simulink model "mmcontrollerVerification_th"  (R2018b)
settings: Solver=ode15s  StartTime=0.0  StopTime=duration_s  MaxStep=5  RelTol=1e-3  AbsTol=1e-3
values from neighbouring files (symbols this model uses):
  ini_euler_ang = [0;ini_pitch;0]    [mmcontrollerVerification_ts.m]
  ini_O_Vcm_o = [0;0;0.0]    [mmcontrollerVerification_ts.m]
  ini_Rcm_o = ini_Rcm_o    [mmcontrollerVerification_ts.m]
undefined symbols (not defined in the file or in its folder): gnd_station, ini_OwB, ini_platform_ang, ini_platform_vel, maxWinchAccel, maxWinchSpeed, R11_g, R1n_cm, R21_g, R2n_cm, R31_g, R3n_cm, rotation_sequence, sim_param, unstretched_l
libraries: thrAttachPtKinematics_ul x6, singleTetherNGreater2_cl x3, winch_ul x3, vrlib x3, eulAng2RotMat_ul x2, combinedController_cl x1, simulink x1, massSpringDamper_ul x1
settings Model: Creator=mcobb  LastModifiedBy=asiddiq2

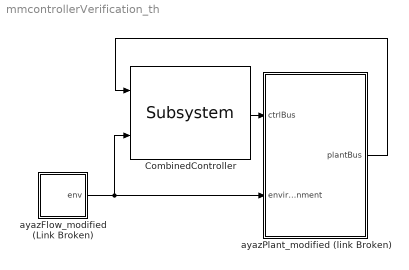
== system mmcontrollerVerification_th ==
  CombinedController : combinedController_cl/Subsystem  a_user=0  b_user=0  phiG_user=0  path_user=0  S_user=0
  ayazFlow_modified (Link Broken) : Subsystem
  ayazPlant_modified (link Broken) : Subsystem
  wires:
  CombinedController/1 -> ayazPlant_modified (link Broken)/1(ctrlBus)
  ayazPlant_modified (link Broken)/1(plantBus) -> CombinedController/1
  ayazFlow_modified (Link Broken)/1(env) -> CombinedController/2, ayazPlant_modified (link Broken)/2(environment)

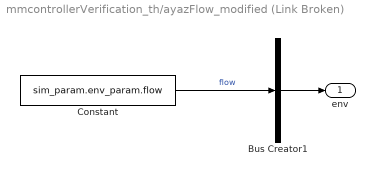
== system mmcontrollerVerification_th/ayazFlow_modified (Link Broken) ==
  Bus Creator1 : BusCreator  Inputs=1  OutDataTypeStr=Bus: envBus
  Constant : Constant  Value=sim_param.env_param.flow
  env : Outport  OutDataTypeStr=Bus: envBus
  wires:
  Constant/1 -> Bus Creator1/1  "flow"
  Bus Creator1/1 -> env/1

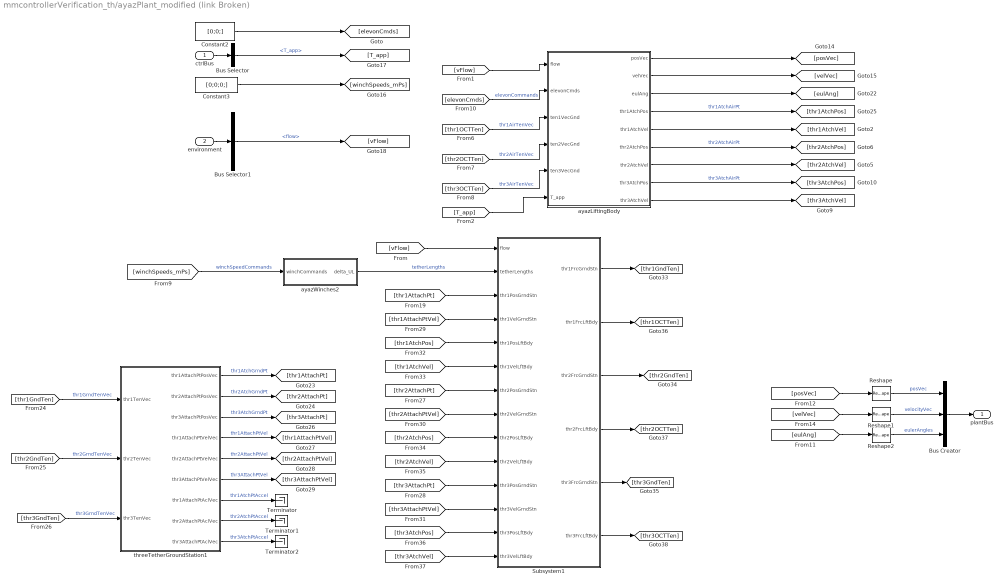
== system mmcontrollerVerification_th/ayazPlant_modified (link Broken) ==
  ctrlBus : Inport  OutDataTypeStr=Bus: ctrlBus
  environment : Inport  Port=2  OutDataTypeStr=Bus: envBus
  Bus Creator : BusCreator  Inputs=3  OutDataTypeStr=Bus: plantBus
  Bus Selector : BusSelector  OutputSignals=T_app
  Bus Selector1 : BusSelector  OutputSignals=flow
  Constant2 : Constant  Value=[0;0;]
  Constant3 : Constant  Value=[0;0;0;]
  Reshape : Reshape  OutputDimensionality=Column vector (2-D)
  Reshape1 : Reshape  OutputDimensionality=Column vector (2-D)
  Reshape2 : Reshape  OutputDimensionality=Column vector (2-D)
  Subsystem1 : Subsystem
  Terminator : Terminator
  Terminator1 : Terminator
  Terminator2 : Terminator
  ayazLiftingBody : Subsystem
  ayazWinches2 : Subsystem  mask{maxSpeed=maxWinchSpeed, maxAccel=maxWinchAccel, timeConst=1, tetherLengths=unstretched_l}
      mask prompts: maxSpeed "Winch Max Speed"; maxAccel "Winch Max Acceleration"; timeConst "Winch Time Constant"; tetherLengths "Initial tether lengths"
  threeTetherGroundStation1 : Subsystem  mask{fixed=1, J=sim_param.platform_param.platform_Izz, b=sim_param.platform_param.platform_damping, posVec=[0 0 0], thr1AttachPt=sim_param.tether_imp_nodes.R11_g, thr2AttachPt=sim_param.tether_imp_nodes.R21_g, thr3AttachPt=sim_param.tether_imp_nodes.R31_g, initAngPos=ini_platform_ang, initAngVel=ini_platform_vel}
      mask prompts: fixed "Free Spin Enable (==0 -> No Rotation, ~=0 -> Free Spinning)"; J "Rotational Inertia"; b "Damping coefficient"; posVec "Position Vector"; thr1AttachPt "Tether 1"; thr2AttachPt "Tether 2"; thr3AttachPt "Tether 3"; initAngPos "Initial angle"; initAngVel "Inital angular velocity"
      mask DialogControl Container5 Prompt: Physical Parameters
      mask DialogControl Container3 Prompt: Tether attachment position vectors: platform frame
      mask DialogControl Container4 Prompt: Initial conditions
  plantBus : Outport  OutDataTypeStr=Bus: plantBus
  wires:
  [eulAng] -> Reshape2/1
  [velVec] -> Reshape1/1
  [posVec] -> Reshape/1
  Subsystem1/5(thr3FrcGrndStn) -> [thr3GndTen]
  Subsystem1/6(thr3FrcLftBdy) -> [thr3OCTTen]
  Subsystem1/4(thr2FrcLftBdy) -> [thr2OCTTen]
  Subsystem1/3(thr2FrcGrndStn) -> [thr2GndTen]
  Subsystem1/2(thr1FrcLftBdy) -> [thr1OCTTen]
  Subsystem1/1(thr1FrcGrndStn) -> [thr1GndTen]
  [thr1AtchVel] -> Subsystem1/6(thr1VelLftBdy)
  [thr2AtchPos] -> Subsystem1/9(thr2PosLftBdy)
  [thr2AtchVel] -> Subsystem1/10(thr2VelLftBdy)
  [thr3AtchPos] -> Subsystem1/13(thr3PosLftBdy)
  [thr3AtchVel] -> Subsystem1/14(thr3VelLftBdy)
  [thr1AtchPos] -> Subsystem1/5(thr1PosLftBdy)
  [thr1AttachPtVel] -> Subsystem1/4(thr1VelGrndStn)
  [thr2AttachPtVel] -> Subsystem1/8(thr2VelGrndStn)
  [thr3AttachPtVel] -> Subsystem1/12(thr3VelGrndStn)
  [thr3AttachPt] -> Subsystem1/11(thr3PosGrndStn)
  [thr2AttachPt] -> Subsystem1/7(thr2PosGrndStn)
  [thr1AttachPt] -> Subsystem1/3(thr1PosGrndStn)
  [vFlow] -> Subsystem1/1(flow)
  threeTetherGroundStation1/7(thr1AttachPtAclVec) -> Terminator/1  "thr1AtchPtAccel"
  [thr1GndTen] -> threeTetherGroundStation1/1(thr1TenVec)  "thr1GrndTenVec"
  [thr3GndTen] -> threeTetherGroundStation1/3(thr3TenVec)  "thr3GrndTenVec"
  [winchSpeeds_mPs] -> ayazWinches2/1(winchCommands)  "winchSpeedCommands"
  [thr2GndTen] -> threeTetherGroundStation1/2(thr2TenVec)  "thr2GrndTenVec"
  ayazWinches2/1(delta_UL) -> Subsystem1/2(tetherLengths)  "tetherLengths"
  threeTetherGroundStation1/1(thr1AttachPtPosVec) -> [thr1AttachPt]  "thr1AtchGrndPt"
  threeTetherGroundStation1/3(thr3AttachPtPosVec) -> [thr3AttachPt]  "thr3AtchGrndPt"
  threeTetherGroundStation1/2(thr2AttachPtPosVec) -> [thr2AttachPt]  "thr2AtchGrndPt"
  threeTetherGroundStation1/4(thr1AttachPtVelVec) -> [thr1AttachPtVel]  "thr1AttachPtVel"
  threeTetherGroundStation1/8(thr2AttachPtAclVec) -> Terminator1/1  "thr2AtchPtAccel"
  threeTetherGroundStation1/5(thr2AttachPtVelVec) -> [thr2AttachPtVel]  "thr2AttachPtVel"
  threeTetherGroundStation1/6(thr3AttachPtVelVec) -> [thr3AttachPtVel]  "thr3AttachPtVel"
  threeTetherGroundStation1/9(thr3AttachPtAclVec) -> Terminator2/1  "thr3AtchPtAccel"
  ayazLiftingBody/9(thr3AtchVel) -> [thr3AtchVel]
  ayazLiftingBody/8(thr3AtchPos) -> [thr3AtchPos]  "thr3AtchAirPt"
  ayazLiftingBody/7(thr2AtchVel) -> [thr2AtchVel]
  ayazLiftingBody/6(thr2AtchPos) -> [thr2AtchPos]  "thr2AtchAirPt"
  ayazLiftingBody/5(thr1AtchVel) -> [thr1AtchVel]
  ayazLiftingBody/4(thr1AtchPos) -> [thr1AtchPos]  "thr1AtchAirPt"
  ayazLiftingBody/3(eulAng) -> [eulAng]
  Reshape1/1 -> Bus Creator/2  "velocityVec"
  Reshape2/1 -> Bus Creator/3  "eulerAngles"
  Reshape/1 -> Bus Creator/1  "posVec"
  Bus Creator/1 -> plantBus/1
  Bus Selector/1 -> [T_app]  "<T_app>"
  ctrlBus/1 -> Bus Selector/1
  environment/1 -> Bus Selector1/1
  [elevonCmds] -> ayazLiftingBody/2(elevonCmds)  "elevonCommands"
  [thr3OCTTen] -> ayazLiftingBody/5(ten3VecGnd)  "thr3AirTenVec"
  [thr2OCTTen] -> ayazLiftingBody/4(ten2VecGnd)  "thr2AirTenVec"
  [thr1OCTTen] -> ayazLiftingBody/3(ten1VecGnd)  "thr1AirTenVec"
  [vFlow] -> ayazLiftingBody/1(flow)
  ayazLiftingBody/2(velVec) -> [velVec]
  ayazLiftingBody/1("posVec ") -> [posVec]
  [T_app] -> ayazLiftingBody/6(T_app)
  Constant2/1 -> [elevonCmds]
  Constant3/1 -> [winchSpeeds_mPs]
  Bus Selector1/1 -> [vFlow]  "<flow>"

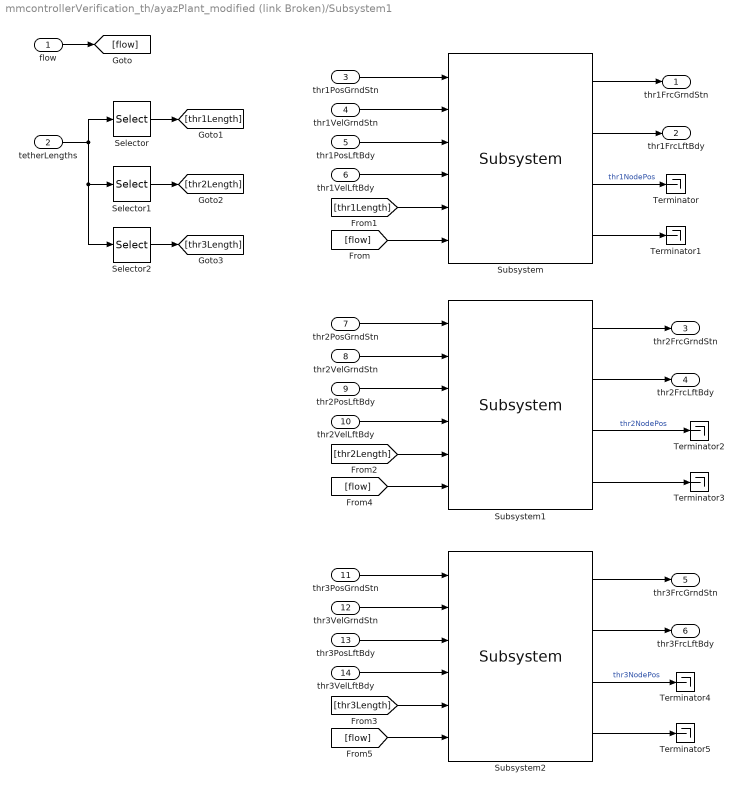
== system mmcontrollerVerification_th/ayazPlant_modified (link Broken)/Subsystem1 ==
  flow : Inport
  tetherLengths : Inport  Port=2
  thr1PosGrndStn : Inport  Port=3
  thr1VelGrndStn : Inport  Port=4
  thr1PosLftBdy : Inport  Port=5
  thr1VelLftBdy : Inport  Port=6
  thr2PosGrndStn : Inport  Port=7
  thr2VelGrndStn : Inport  Port=8
  thr2PosLftBdy : Inport  Port=9
  thr2VelLftBdy : Inport  Port=10
  thr3PosGrndStn : Inport  Port=11
  thr3VelGrndStn : Inport  Port=12
  thr3PosLftBdy : Inport  Port=13
  thr3VelLftBdy : Inport  Port=14
  Selector : Selector  InputPortWidth=3  IndexOptions=Index vector (dialog)  Indices=1  OutputSizes=1
  Selector1 : Selector  InputPortWidth=3  IndexOptions=Index vector (dialog)  Indices=2  OutputSizes=1
  Selector2 : Selector  InputPortWidth=3  IndexOptions=Index vector (dialog)  Indices=3  OutputSizes=1
  Subsystem : singleTetherNGreater2_cl/Subsystem  N=sim_param.N  dia_t=sim_param.tether_param.tether_diameter(1)  E=sim_param.tether_param.tether_youngs  rho_tether=sim_param.tether_param.tether_density+ sim_param.env_param.density  Cd=sim_param.tether_param.CD_cylinder  zeta=sim_param.tether_param.damping_ratio  rho=sim_param.env_param.density  g=sim_param.env_param.grav  mass=sim_param.geom_param.mass  ini_Rn_o=ini_Rcm_o + rotation_sequence(ini_euler_ang)*R1n_cm  ini_R1_o=gnd_station + R11_g
  Subsystem1 : singleTetherNGreater2_cl/Subsystem  N=sim_param.N  dia_t=sim_param.tether_param.tether_diameter(2)  E=sim_param.tether_param.tether_youngs  rho_tether=sim_param.tether_param.tether_density+ sim_param.env_param.density  Cd=sim_param.tether_param.CD_cylinder  zeta=sim_param.tether_param.damping_ratio  rho=sim_param.env_param.density  g=sim_param.env_param.grav  mass=sim_param.geom_param.mass  ini_Rn_o=ini_Rcm_o + rotation_sequence(ini_euler_ang)*R2n_cm  ini_R1_o=gnd_station + R21_g
  Subsystem2 : singleTetherNGreater2_cl/Subsystem  N=sim_param.N  dia_t=sim_param.tether_param.tether_diameter(3)  E=sim_param.tether_param.tether_youngs  rho_tether=sim_param.tether_param.tether_density+ sim_param.env_param.density  Cd=sim_param.tether_param.CD_cylinder  zeta=sim_param.tether_param.damping_ratio  rho=sim_param.env_param.density  g=sim_param.env_param.grav  mass=sim_param.geom_param.mass  ini_Rn_o=ini_Rcm_o + rotation_sequence(ini_euler_ang)*R3n_cm  ini_R1_o=gnd_station + R31_g
  Terminator{,1..5} (6 alike) : Terminator
  thr1FrcGrndStn : Outport
  thr1FrcLftBdy : Outport  Port=2
  thr2FrcGrndStn : Outport  Port=3
  thr2FrcLftBdy : Outport  Port=4
  thr3FrcGrndStn : Outport  Port=5
  thr3FrcLftBdy : Outport  Port=6
  wires:
  Subsystem1/1 -> thr2FrcGrndStn/1
  Subsystem1/2 -> thr2FrcLftBdy/1
  Subsystem1/3 -> Terminator2/1  "thr2NodePos"
  Subsystem1/4 -> Terminator3/1
  Subsystem2/1 -> thr3FrcGrndStn/1
  Subsystem2/2 -> thr3FrcLftBdy/1
  Subsystem2/3 -> Terminator4/1  "thr3NodePos"
  Subsystem2/4 -> Terminator5/1
  Subsystem/4 -> Terminator1/1
  Subsystem/3 -> Terminator/1  "thr1NodePos"
  Subsystem/2 -> thr1FrcLftBdy/1
  Subsystem/1 -> thr1FrcGrndStn/1
  thr3PosGrndStn/1 -> Subsystem2/1
  thr3VelGrndStn/1 -> Subsystem2/2
  thr3PosLftBdy/1 -> Subsystem2/3
  thr3VelLftBdy/1 -> Subsystem2/4
  thr2VelLftBdy/1 -> Subsystem1/4
  thr2PosLftBdy/1 -> Subsystem1/3
  thr2VelGrndStn/1 -> Subsystem1/2
  thr2PosGrndStn/1 -> Subsystem1/1
  [flow] -> Subsystem2/6
  [flow] -> Subsystem1/6
  [thr3Length] -> Subsystem2/5
  [thr2Length] -> Subsystem1/5
  [thr1Length] -> Subsystem/5
  Selector2/1 -> [thr3Length]
  Selector1/1 -> [thr2Length]
  tetherLengths/1 -> Selector2/1, Selector1/1, Selector/1
  Selector/1 -> [thr1Length]
  [flow] -> Subsystem/6
  flow/1 -> [flow]
  thr1PosLftBdy/1 -> Subsystem/3
  thr1VelLftBdy/1 -> Subsystem/4
  thr1VelGrndStn/1 -> Subsystem/2
  thr1PosGrndStn/1 -> Subsystem/1

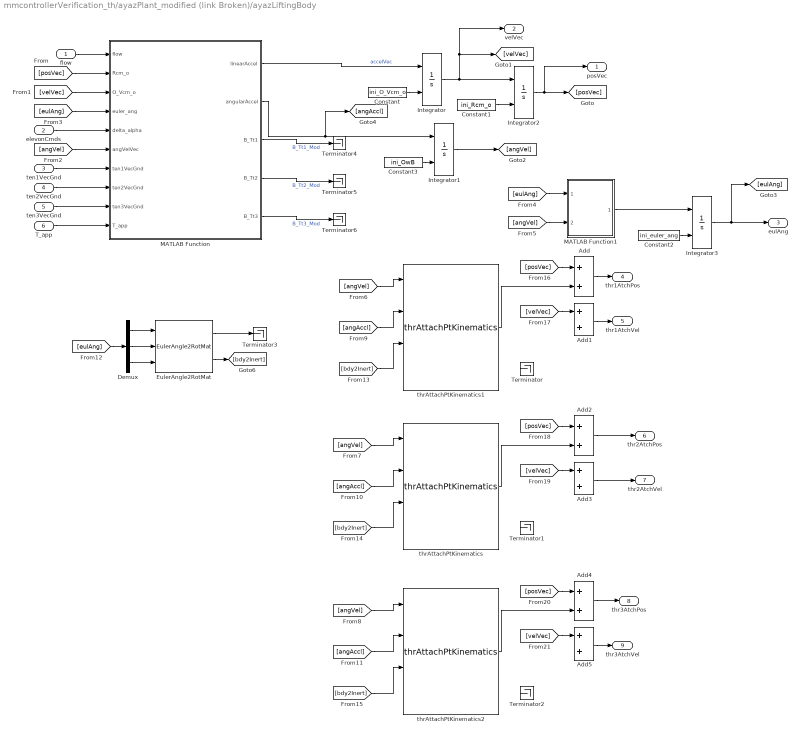
== system mmcontrollerVerification_th/ayazPlant_modified (link Broken)/ayazLiftingBody ==
  flow : Inport
  elevonCmds : Inport  Port=2
  ten1VecGnd : Inport  Port=3
  ten2VecGnd : Inport  Port=4
  ten3VecGnd : Inport  Port=5
  T_app : Inport  Port=6
  Add{,1..5} (6 alike) : Sum
  Constant : Constant  Value=ini_O_Vcm_o
  Constant1 : Constant  Value=ini_Rcm_o
  Constant2 : Constant  Value=ini_euler_ang
  Constant3 : Constant  Value=ini_OwB
  Demux : Demux  Outputs=3
  EulerAngle2RotMat : eulAng2RotMat_ul/EulerAngle2RotMat  SystemSampleTime=-1
  Integrator{,1..3} (4 alike) : Integrator  InitialConditionSource=external
  MATLAB Function : MATLAB Function  TreatAsAtomicUnit=on
  MATLAB Function1 : MATLAB Function  TreatAsAtomicUnit=on
  Terminator{,1..6} (7 alike) : Terminator
  thrAttachPtKinematics : thrAttachPtKinematics_ul/thrAttachPtKinematics  atchPts=gndStnMmtArms
  thrAttachPtKinematics1 : thrAttachPtKinematics_ul/thrAttachPtKinematics  atchPts=gndStnMmtArms
  thrAttachPtKinematics2 : thrAttachPtKinematics_ul/thrAttachPtKinematics  atchPts=gndStnMmtArms
  "posVec " : Outport
  velVec : Outport  Port=2
  eulAng : Outport  Port=3
  thr1AtchPos : Outport  Port=4
  thr1AtchVel : Outport  Port=5
  thr2AtchPos : Outport  Port=6
  thr2AtchVel : Outport  Port=7
  thr3AtchPos : Outport  Port=8
  thr3AtchVel : Outport  Port=9
  wires:
  MATLAB Function/5(B_Tt3) -> Terminator6/1  "B_Tt3_Mod"
  MATLAB Function/4(B_Tt2) -> Terminator5/1  "B_Tt2_Mod"
  MATLAB Function/3(B_Tt1) -> Terminator4/1  "B_Tt1_Mod"
  Add4/1 -> thr3AtchPos/1
  Add5/1 -> thr3AtchVel/1
  [velVec] -> Add5/1
  [posVec] -> Add4/1
  ? -> Add5/2
  thrAttachPtKinematics2/1 -> Add4/2
  Add3/1 -> thr2AtchVel/1
  Add2/1 -> thr2AtchPos/1
  thrAttachPtKinematics/1 -> Add2/2
  ? -> Add3/2
  [posVec] -> Add2/1
  [velVec] -> Add3/1
  Add1/1 -> thr1AtchVel/1
  [velVec] -> Add1/1
  [posVec] -> Add/1
  Add/1 -> thr1AtchPos/1
  EulerAngle2RotMat/1 -> Terminator3/1
  ? -> Terminator2/1
  ? -> Terminator1/1
  ? -> Terminator/1
  ? -> Add1/2
  thrAttachPtKinematics1/1 -> Add/2
  [bdy2Inert] -> thrAttachPtKinematics2/3
  [bdy2Inert] -> thrAttachPtKinematics/3
  [bdy2Inert] -> thrAttachPtKinematics1/3
  EulerAngle2RotMat/2 -> [bdy2Inert]
  Demux/3 -> EulerAngle2RotMat/3
  Demux/1 -> EulerAngle2RotMat/1
  Demux/2 -> EulerAngle2RotMat/2
  [eulAng] -> Demux/1
  [angAccl] -> thrAttachPtKinematics2/2
  [angAccl] -> thrAttachPtKinematics/2
  [angAccl] -> thrAttachPtKinematics1/2
  [angVel] -> thrAttachPtKinematics2/1
  [angVel] -> thrAttachPtKinematics/1
  [angVel] -> thrAttachPtKinematics1/1
  MATLAB Function1/1(eulAngDeriv) -> Integrator3/1
  [angVel] -> MATLAB Function1/2(angVel)
  [eulAng] -> MATLAB Function1/1(eulAng)
  Constant3/1 -> Integrator1/2
  Constant2/1 -> Integrator3/2
  Constant1/1 -> Integrator2/2
  Constant/1 -> Integrator/2
  elevonCmds/1 -> MATLAB Function/5(delta_alpha)
  flow/1 -> MATLAB Function/1(flow)
  MATLAB Function/1(linearAccel) -> Integrator/1  "accelVec"
  MATLAB Function/2(angularAccel) -> Integrator1/1, [angAccl]
  Integrator1/1 -> [angVel]
  Integrator/1 -> Integrator2/1, [velVec], velVec/1
  Integrator2/1 -> [posVec], "posVec "/1
  [posVec] -> MATLAB Function/2(Rcm_o)
  [velVec] -> MATLAB Function/3(O_Vcm_o)
  Integrator3/1 -> [eulAng], eulAng/1
  [angVel] -> MATLAB Function/6(angVelVec)
  [eulAng] -> MATLAB Function/4(euler_ang)
  ten1VecGnd/1 -> MATLAB Function/7(ten1VecGnd)
  ten2VecGnd/1 -> MATLAB Function/8(ten2VecGnd)
  ten3VecGnd/1 -> MATLAB Function/9(ten3VecGnd)
  T_app/1 -> MATLAB Function/10(T_app)

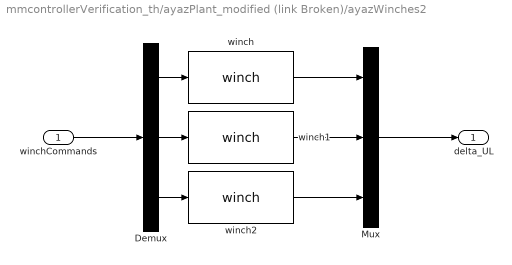
== system mmcontrollerVerification_th/ayazPlant_modified (link Broken)/ayazWinches2 ==
  winchCommands : Inport
  Demux : Demux  Outputs=3
  Mux : Mux  Inputs=3
  winch : winch_ul/winch  initLength=tetherLengths(1)  maxSpd=maxSpeed(1)  tau=timeConst  maxAccl=maxAccel
  winch1 : winch_ul/winch  initLength=tetherLengths(2)  maxSpd=maxSpeed(2)  tau=timeConst  maxAccl=maxAccel
  winch2 : winch_ul/winch  initLength=tetherLengths(3)  maxSpd=maxSpeed(3)  tau=timeConst  maxAccl=maxAccel
  delta_UL : Outport
  wires:
  winch2/1 -> Mux/3
  winch/1 -> Mux/1
  winch1/1 -> Mux/2
  winchCommands/1 -> Demux/1
  Demux/3 -> winch2/1
  Demux/2 -> winch1/1
  Mux/1 -> delta_UL/1
  Demux/1 -> winch/1

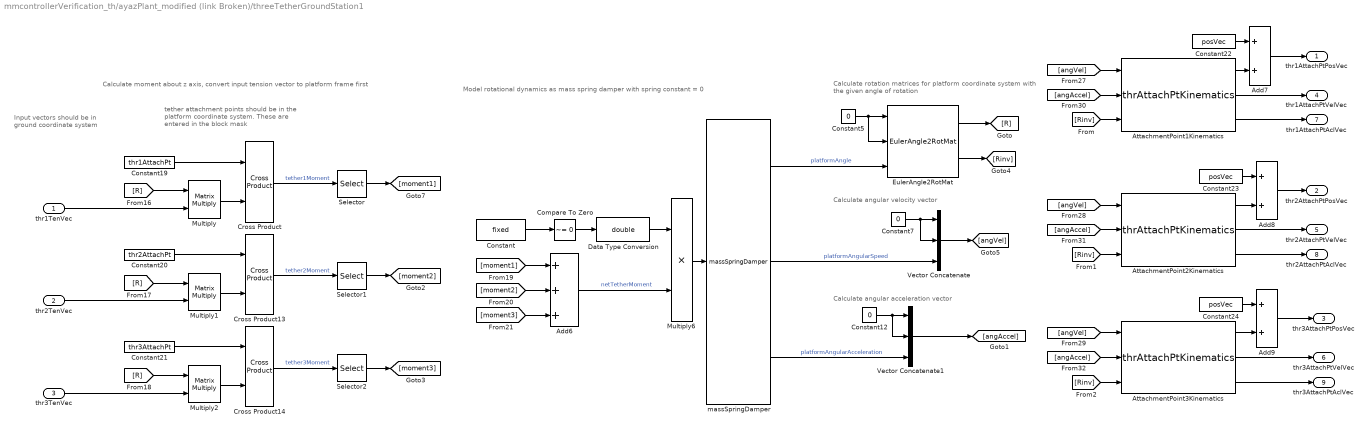
== system mmcontrollerVerification_th/ayazPlant_modified (link Broken)/threeTetherGroundStation1 ==
  note: Model rotational dynamics as mass spring damper with
      | spring constant = 0
  note: Calculate moment about z axis, convert input tension vector to platform frame first
  note: tether attachment points should be in
      | the platform coordinate system.  These
      | are entered in the block mask
  note: Calculate angular velocity vector
  note: Input vectors should be in
      | ground coordinate system
  note: Calculate rotation matrices for platform coordinate
      | system with the given angle of rotation
  note: Calculate angular acceleration vector
  thr1TenVec : Inport
  thr2TenVec : Inport  Port=2
  thr3TenVec : Inport  Port=3
  Add6 : Sum  Inputs=+++
  Add7 : Sum
  Add8 : Sum
  Add9 : Sum
  AttachmentPoint1Kinematics : thrAttachPtKinematics_ul/thrAttachPtKinematics  theAtchPosVec=thr1AttachPt
  AttachmentPoint2Kinematics : thrAttachPtKinematics_ul/thrAttachPtKinematics  theAtchPosVec=thr2AttachPt
  AttachmentPoint3Kinematics : thrAttachPtKinematics_ul/thrAttachPtKinematics  theAtchPosVec=thr3AttachPt
  Compare To Zero : simulink/Logic and Bit Operations/Compare To Zero  relop=~=  OutDataTypeStr=boolean
  Constant : Constant  Value=fixed
  Constant12 : Constant  Value=0
  Constant19 : Constant  Value=thr1AttachPt
  Constant20 : Constant  Value=thr2AttachPt
  Constant21 : Constant  Value=thr3AttachPt
  Constant22 : Constant  Value=posVec
  Constant23 : Constant  Value=posVec
  Constant24 : Constant  Value=posVec
  Constant5 : Constant  Value=0
  Constant7 : Constant  Value=0
  Cross Product : vrlib/Utilities/Cross Product
      settings: SourceProductBaseCode=VR
  Cross Product13 : vrlib/Utilities/Cross Product
      settings: SourceProductBaseCode=VR
  Cross Product14 : vrlib/Utilities/Cross Product
      settings: SourceProductBaseCode=VR
  Data Type Conversion : DataTypeConversion  OutDataTypeStr=double
  EulerAngle2RotMat : eulAng2RotMat_ul/EulerAngle2RotMat  SystemSampleTime=-1
  Multiply : Product  Multiplication=Matrix(*)
  Multiply1 : Product  Multiplication=Matrix(*)
  Multiply2 : Product  Multiplication=Matrix(*)
  Multiply6 : Product
  Selector : Selector  InputPortWidth=3  IndexOptions=Index vector (dialog)  Indices=3  OutputSizes=1
  Selector1 : Selector  InputPortWidth=3  IndexOptions=Index vector (dialog)  Indices=3  OutputSizes=1
  Selector2 : Selector  InputPortWidth=3  IndexOptions=Index vector (dialog)  Indices=3  OutputSizes=1
  Vector Concatenate : Concatenate  NumInputs=3
  Vector Concatenate1 : Concatenate  NumInputs=3
  massSpringDamper : massSpringDamper_ul/massSpringDamper  m=J  b=b  k=0  x0=initAngPos  xDot0=initAngVel
  thr1AttachPtPosVec : Outport
  thr2AttachPtPosVec : Outport  Port=2
  thr3AttachPtPosVec : Outport  Port=3
  thr1AttachPtVelVec : Outport  Port=4
  thr2AttachPtVelVec : Outport  Port=5
  thr3AttachPtVelVec : Outport  Port=6
  thr1AttachPtAclVec : Outport  Port=7
  thr2AttachPtAclVec : Outport  Port=8
  thr3AttachPtAclVec : Outport  Port=9
  wires:
  Add9/1 -> thr3AttachPtPosVec/1
  Constant24/1 -> Add9/1
  Add8/1 -> thr2AttachPtPosVec/1
  Constant23/1 -> Add8/1
  Constant22/1 -> Add7/1
  Add7/1 -> thr1AttachPtPosVec/1
  [angAccel] -> AttachmentPoint3Kinematics/2
  [angAccel] -> AttachmentPoint2Kinematics/2
  [angAccel] -> AttachmentPoint1Kinematics/2
  [angVel] -> AttachmentPoint3Kinematics/1
  [angVel] -> AttachmentPoint2Kinematics/1
  [angVel] -> AttachmentPoint1Kinematics/1
  AttachmentPoint3Kinematics/3 -> thr3AttachPtAclVec/1
  AttachmentPoint3Kinematics/2 -> thr3AttachPtVelVec/1
  AttachmentPoint2Kinematics/3 -> thr2AttachPtAclVec/1
  AttachmentPoint2Kinematics/2 -> thr2AttachPtVelVec/1
  AttachmentPoint2Kinematics/1 -> Add8/2
  AttachmentPoint3Kinematics/1 -> Add9/2
  AttachmentPoint1Kinematics/2 -> thr1AttachPtVelVec/1
  AttachmentPoint1Kinematics/3 -> thr1AttachPtAclVec/1
  AttachmentPoint1Kinematics/1 -> Add7/2
  [Rinv] -> AttachmentPoint3Kinematics/3
  [Rinv] -> AttachmentPoint2Kinematics/3
  [Rinv] -> AttachmentPoint1Kinematics/3
  Vector Concatenate1/1 -> [angAccel]
  Add6/1 -> Multiply6/2  "netTetherMoment"
  Data Type Conversion/1 -> Multiply6/1
  Multiply6/1 -> massSpringDamper/1
  Selector1/1 -> [moment2]
  Constant19/1 -> Cross Product/1
  [R] -> Multiply2/1
  [R] -> Multiply1/1
  [moment1] -> Add6/1
  [R] -> Multiply/1
  [moment3] -> Add6/3
  Cross Product14/1 -> Selector2/1  "tether3Moment"
  Cross Product/1 -> Selector/1  "tether1Moment"
  Constant21/1 -> Cross Product14/1
  Cross Product13/1 -> Selector1/1  "tether2Moment"
  Constant20/1 -> Cross Product13/1
  Multiply/1 -> Cross Product/2
  Multiply1/1 -> Cross Product13/2
  Multiply2/1 -> Cross Product14/2
  Selector/1 -> [moment1]
  [moment2] -> Add6/2
  Selector2/1 -> [moment3]
  thr3TenVec/1 -> Multiply2/2
  thr2TenVec/1 -> Multiply1/2
  thr1TenVec/1 -> Multiply/2
  Constant12/1 -> Vector Concatenate1/2, Vector Concatenate1/1
  massSpringDamper/3 -> Vector Concatenate1/3  "platformAngularAcceleration"
  Compare To Zero/1 -> Data Type Conversion/1
  Constant/1 -> Compare To Zero/1
  massSpringDamper/2 -> Vector Concatenate/3  "platformAngularSpeed"
  massSpringDamper/1 -> EulerAngle2RotMat/3  "platformAngle"
  Vector Concatenate/1 -> [angVel]
  Constant7/1 -> Vector Concatenate/2, Vector Concatenate/1
  EulerAngle2RotMat/2 -> [Rinv]
  EulerAngle2RotMat/1 -> [R]
  Constant5/1 -> EulerAngle2RotMat/1, EulerAngle2RotMat/2

== matlab function mmcontrollerVerification_th/ayazPlant_modified (link Broken)/ayazLiftingBody/MATLAB Function ==
  data: sim_param parameter; flow input; linearAccel output size=[3 1]; Rcm_o input; O_Vcm_o input; euler_ang input; delta_alpha input; angVelVec input; angularAccel output size=[3 1]; ten1VecGnd input; ten2VecGnd input; ten3VecGnd input; B_Tt1 output; B_Tt2 output; B_Tt3 output; T_app input
function [linearAccel, angularAccel,B_Tt1,B_Tt2,B_Tt3] = B_F_and_T_aero(sim_param,flow,Rcm_o,...
    O_Vcm_o,euler_ang,delta_alpha,angVelVec,ten1VecGnd,ten2VecGnd,...
    ten3VecGnd,T_app)
%% extracting values from sim parameters structure
N = sim_param.N;

env_param = sim_param.env_param;
geom_param = sim_param.geom_param;
aero_param = sim_param.aero_param;
turbine_param = sim_param.turbine_param;
tether_param = sim_param.tether_param;
tether_imp_nodes = sim_param.tether_imp_nodes;


m = geom_param.mass;
m_added = geom_param.m_added;
g = env_param.grav;
% rho = env_param.density;

% CD_cylinder = tether_param.CD_cylinder;
% tether_youngs = tether_param.tether_youngs;


Rcb_cm = geom_param.center_of_buoy;
% Rac_cm = geom_param.aero_center;
% R1turb_cm = turbine_param.R1turb_cm;
% R2turb_cm = turbine_param.R2turb_cm;


% Rvs_cm = aero_param.Rvs_cm;

R1n_cm = tether_imp_nodes.R1n_cm;
R2n_cm = tether_imp_nodes.R2n_cm;
R3n_cm = tether_imp_nodes.R3n_cm;

% R11_g = tether_imp_nodes.R11_g;
% R21_g = tether_imp_nodes.R21_g;
% R31_g = tether_imp_nodes.R31_g;


% calculate tether masses and spring stiffness
% tether_density = tether_param.tether_density;
% tether_dia = tether_param.tether_diameter;
% zeta = tether_param.damping_ratio;

% tether_masses = ((tether_density*(pi/4)).*tether_dia.^2).*unstretched_l;

%% force calculations
% buoyancy force in the ko direction
fz_buoy = geom_param.F_buoy;

% buoyancy force in the O frame
O_F_buoy = [0;0;fz_buoy];

% gravity force in the ko direction
fz_grav = -m*g;

% gravity force in the O frame
O_F_grav = [0;0;fz_grav];

% calculate aerodynamic forces on the lifting body
aero_F = B_F_and_T_aero(sim_param,flow,Rcm_o,O_Vcm_o,euler_ang,delta_alpha);

B_F_aero_mw = aero_F.B_F_aero_mw;
B_F_aero_VS = aero_F.B_F_aero_VS;
B_F_turb1 = aero_F.B_F_turb1;
B_F_turb2 = aero_F.B_F_turb2;

B_T_aero_mw = aero_F.B_T_aero_mw;
B_T_aero_VS = aero_F.B_T_aero_VS;
B_T_aero_turb = aero_F.B_T_aero_turb;


O_F_aero_mw = oCb*B_F_aero_mw;
O_F_aero_VS = oCb*B_F_aero_VS;
O_F_turb1 = oCb*B_F_turb1;
O_F_turb2 = oCb*B_F_turb2;

% %% forces acting on the center of mass
O_F_ext = O_F_buoy + O_F_grav + O_F_aero_mw + O_F_aero_VS + O_F_turb1 + O_F_turb2 +...
    ten1VecGnd + ten2VecGnd + ten3VecGnd;

mass_matrix = [1/(m+m_added(1)) 0 0;0 1/(m+m_added(2)) 0;0 0 1/(m+m_added(3))];


linearAccel = oCb*(mass_matrix*bCo*O_F_ext);
B_T_buoy = cross(Rcb_cm,(bCo*O_F_buoy));
% torque due to gravity about CM
B_T_grav = [0;0;0];

% torque due to the three tethers in the B frame
B_Tt1 = cross(R1n_cm,(bCo*ten1VecGnd));
B_Tt2 = cross(R2n_cm,(bCo*ten2VecGnd));
B_Tt3 = cross(R3n_cm,(bCo*ten3VecGnd));

B_T_ext = B_T_buoy + B_T_grav + B_T_aero_mw + B_T_aero_VS + B_T_aero_turb + ...
    B_Tt1 + B_Tt2 + B_Tt3;

Tx = B_T_ext(1)+T_app(1);
Ty = B_T_ext(2)+T_app(2);
Tz = B_T_ext(3)+T_app(3);

wx = angVelVec(1);
wy = angVelVec(2);
wz = angVelVec(3);

MI = sim_param.geom_param.MI;
Ixx = MI(1,1);
Iyy = MI(2,2);
Izz = MI(3,3);
Izz_added = sim_param.geom_param.Izz_added;

angularAccel = [...
    (1/Ixx)*(Tx + (Iyy - Izz)*wy*wz);...
    (1/Iyy)*(Ty + (Izz - Ixx)*wx*wz);...
    (1/(Izz+Izz_added))*(Tz + (Ixx - Iyy)*wx*wy)];

end

== matlab function mmcontrollerVerification_th/ayazPlant_modified (link Broken)/ayazLiftingBody/MATLAB Function1 ==
  data: eulAng input; eulAngDeriv output; angVel input
function eulAngDeriv = fcn(eulAng,angVel)

wx = angVel(1);
wy = angVel(2);
wz = angVel(3);

ph = eulAng(1);
th = eulAng(2);

eulAngDeriv = zeros(3,1);
eulAngDeriv(1) = wx + sin(ph)*tan(th)*wy + cos(ph)*tan(th)*wz;
eulAngDeriv(2) = cos(ph)*wy - sin(ph)*wz;
eulAngDeriv(3) = sec(th)*sin(ph)*wy + cos(ph)*sec(th)*wz;
